simulink model "untitled5"  (R2022a)
settings: Solver=VariableStepAuto  StartTime=0.0  StopTime=100  RelTol=1e-3
undefined symbols (not defined in the file): DiscIntNeverNeededParam
settings Model: Creator=mluser  LastModifiedBy=mluser
settings ModelReferenceCC: EnableRefExpFcnMdlSchedulingChecks=off
settings RTWCC: Description=Generic Real-Time Target

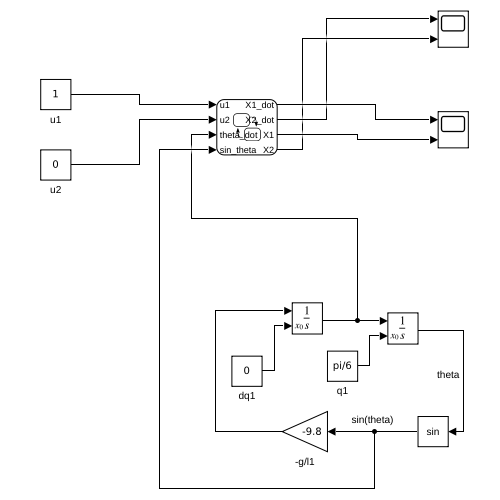
[thumbnail: Simulink's stored preview of the top-level diagram]
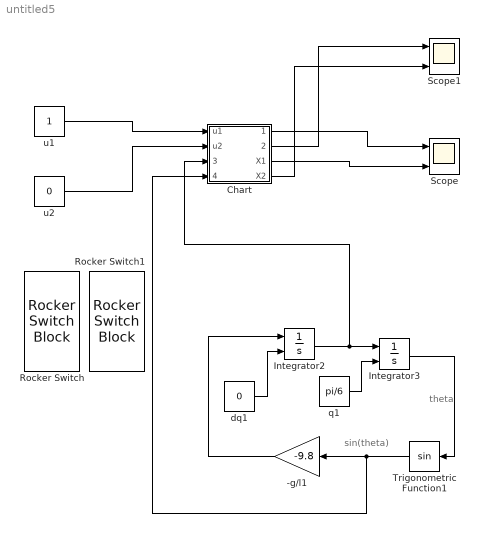
== system untitled5 ==
  note: theta
  note: sin(theta)
  -g/l1 : Gain  Gain=-9.8
  Chart : Stateflow chart  TreatAsAtomicUnit=on
  Integrator2 : Integrator  InitialConditionSource=external
  Integrator3 : Integrator  InitialConditionSource=external
  Rocker Switch : RockerSwitchBlock
      settings: Values={{'Off', 'On'}, [0 1]}
  Rocker Switch1 : RockerSwitchBlock
      settings: Values={{'Off', 'On'}, [0 1]}
  Scope : Scope  NumInputPorts=2
  Scope1 : Scope  NumInputPorts=2
  Trigonometric Function1 : Trigonometry
  dq1 : Constant  Value=0
  q1 : Constant  Value=pi/6
  u1 : Constant
  u2 : Constant  Value=0
  wires:
  Chart/1(X1_dot) -> Scope/1
  u1/1 -> Chart/1(u1)
  u2/1 -> Chart/2(u2)
  Trigonometric Function1/1 -> Chart/4(sin_theta), -g/l1/1
  Integrator3/1 -> Trigonometric Function1/1
  Integrator2/1 -> Chart/3(theta_dot), Integrator3/1
  -g/l1/1 -> Integrator2/1
  dq1/1 -> Integrator2/2
  q1/1 -> Integrator3/2
  Chart/3(X1) -> Scope/2
  Chart/2(X2_dot) -> Scope1/1
  Chart/4(X2) -> Scope1/2

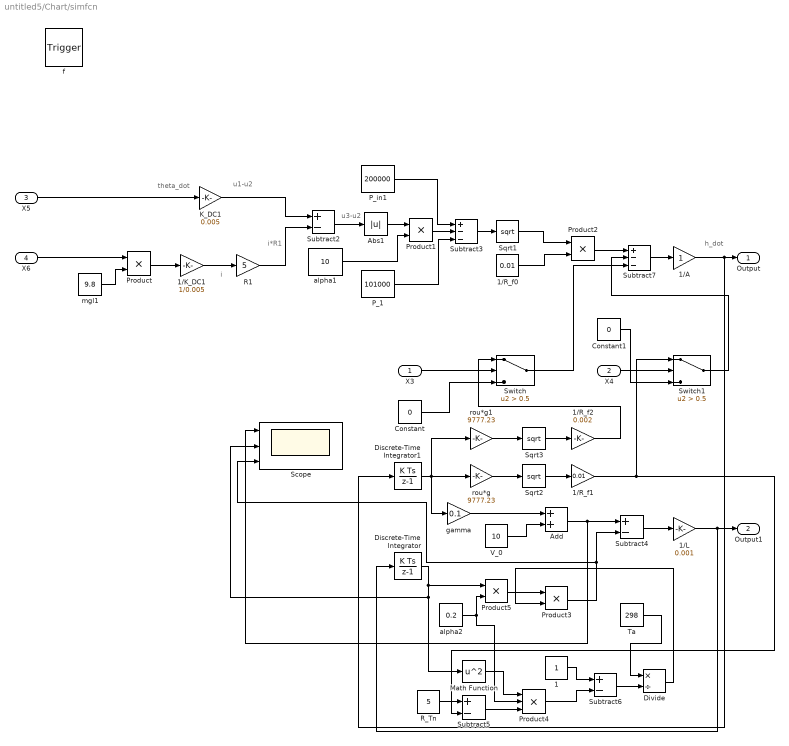
== system untitled5/Chart/simfcn ==
  note: u1-u2
  note: i*R1
  note: u3-u2
  note: theta_dot
  note: h_dot
  note: i
  X3 : Inport  OutDataTypeStr=double  PortDimensions=1
  X4 : Inport  Port=2  OutDataTypeStr=double  PortDimensions=1
  X5 : Inport  Port=3  OutDataTypeStr=double  PortDimensions=1
  X6 : Inport  Port=4  OutDataTypeStr=double  PortDimensions=1
  f : TriggerPort  TriggerType=function-call  VariantControl=(inherit)
      settings: CopyFcn=Stateflow.SLINSF.SimulinkMan.removeBlockPreDeleteFcn  PreDeleteFcn=Stateflow.SLINSF.SimulinkMan.unsafePredeleteFcn
  1 : Constant
  1/A : Gain
  1/K_DC1 : Gain  Gain=1/0.005
  1/L : Gain  Gain=0.001
  1/R_f0 : Constant  Value=0.01
  1/R_f1 : Gain  Gain=0.01
  1/R_f2 : Gain  Gain=0.002
  Abs1 : Abs  SaturateOnIntegerOverflow=off
  Add : Sum
  Constant : Constant  Value=0
  Constant1 : Constant  Value=0
  Discrete-Time Integrator : DiscreteIntegrator  SampleTime=-1  ICPrevOutput=DiscIntNeverNeededParam  ICPrevScaledInput=DiscIntNeverNeededParam
  Discrete-Time Integrator1 : DiscreteIntegrator  SampleTime=-1  ICPrevOutput=DiscIntNeverNeededParam  ICPrevScaledInput=DiscIntNeverNeededParam
  Divide : Product  Inputs=*/
  K_DC1 : Gain  Gain=0.005
  Math Function : Math  Operator=square
  P_1 : Constant  Value=101000
  P_in1 : Constant  Value=200000
  Product{,1..3,5} (5 alike) : Product
  Product4 : Product  Inputs=3
  R1 : Gain  Gain=5
  R_Tn : Constant  Value=5
  Scope : Scope  NumInputPorts=5
  Sqrt1 : Sqrt
  Sqrt2 : Sqrt
  Sqrt3 : Sqrt
  Subtract{2,4..6} (4 alike) : Sum  Inputs=+-
  Subtract3 : Sum  Inputs=+--
  Subtract7 : Sum  Inputs=+--
  Switch : Switch  Criteria=u2 > Threshold  Threshold=0.5  SaturateOnIntegerOverflow=off  InputSameDT=off
  Switch1 : Switch  Criteria=u2 > Threshold  Threshold=0.5  SaturateOnIntegerOverflow=off  InputSameDT=off
  Ta : Constant  Value=298
  V_0 : Constant  Value=10
  alpha1 : Constant  Value=10
  alpha2 : Constant  Value=0.2
  gamma : Gain  Gain=0.1
  mgl1 : Constant  Value=9.8
  rou*g : Gain  Gain=9777.23
  rou*g1 : Gain  Gain=9777.23
  Output : Outport
  Output1 : Outport  Port=2
  wires:
  Switch/1 -> Subtract7/3
  Math Function/1 -> Product4/1
  gamma/1 -> Add/1
  1/L/1 -> Discrete-Time Integrator/1, Output1/1
  Sqrt3/1 -> 1/R_f2/1
  X3/1 -> Switch/2
  rou*g1/1 -> Sqrt3/1
  Product2/1 -> Subtract7/1
  Abs1/1 -> Product1/1
  Product1/1 -> Subtract3/2
  alpha1/1 -> Product1/2
  1/R_f1/1 -> Switch1/1, Subtract5/2
  Discrete-Time Integrator/1 -> Math Function/1, Scope/3, Product5/1
  Subtract5/1 -> Product4/3
  Product3/1 -> Subtract4/2, Scope/5
  R_Tn/1 -> Subtract5/1
  Constant/1 -> Switch/3
  Sqrt1/1 -> Product2/1
  Product/1 -> 1/K_DC1/1
  Subtract4/1 -> 1/L/1
  alpha2/1 -> Product5/2, Product4/2
  Discrete-Time Integrator1/1 -> rou*g1/1, gamma/1, rou*g/1
  R1/1 -> Subtract2/2
  Switch1/1 -> Subtract7/2
  Subtract7/1 -> 1/A/1
  mgl1/1 -> Product/2
  P_in1/1 -> Subtract3/1
  Divide/1 -> Product3/2
  rou*g/1 -> Sqrt2/1
  Sqrt2/1 -> 1/R_f1/1
  1/R_f0/1 -> Product2/2
  Constant1/1 -> Switch1/3
  K_DC1/1 -> Subtract2/1
  Add/1 -> Scope/1, Subtract4/1
  Ta/1 -> Divide/1
  1/1 -> Subtract6/1
  Product4/1 -> Subtract6/2
  V_0/1 -> Add/2
  Product5/1 -> Product3/1
  1/R_f2/1 -> Switch/1
  Subtract6/1 -> Divide/2
  1/K_DC1/1 -> R1/1
  P_1/1 -> Subtract3/3
  Subtract3/1 -> Sqrt1/1
  X4/1 -> Switch1/2
  X5/1 -> K_DC1/1
  X6/1 -> Product/1
  Subtract2/1 -> Abs1/1
  1/A/1 -> Discrete-Time Integrator1/1, Output/1

== stateflow chart untitled5/Chart ==
  state [Output,Output1] = simfcn(X3,X4,X5,X6) [function]
  state state
    du:
    [Output,Output1] = simfcn(u1,u2,theta_dot,sin_theta);
    X1_dot=Output;
    X2_dot=Output1;
  (default) -> state : {X1=0;
      | X2=0;}
  data: X3 function_input double size=1; X4 function_input double size=1; Output function_output; Output1 function_output; X5 function_input double size=1; X6 function_input double size=1; u1 input; u2 input; X1_dot output; X2_dot output; Output1 local; Output local; X1 output; X2 output; theta_dot input; sin_theta input
